simulink model "chris_3R_hsv_all_primitives"  (R2024b)
settings: Solver=FixedStepDiscrete  StartTime=0.0  StopTime=30  FixedStep=0.1  MaxStep=0.1  RelTol=1e-3
libraries: neural x110, realtime_pacer_lib x1, simulink x1
(part 2 of 7)

== system chris_3R_hsv_all_primitives/Cluster_Controller_HSV_steepest_descent/3_robot HSV to vector ==
  Sat : Inport
  Robot_1_pose : Inport  Port=2
  robot_2_pose : Inport  Port=3
  robot_3_pose : Inport  Port=4
  Constant2 : Constant  Value=0
  Demux{,1..3} (4 alike) : Demux  Outputs=3
  Desired_velocities_new_primitve : ToWorkspace  VariableName=desired_velocities_gradient_descent  SampleTime=-1
  MATLAB Function : MATLAB Function  TreatAsAtomicUnit=on
  Scope : Scope  NumInputPorts=2
  Scope1 : Scope  NumInputPorts=2
  Scope2 : Scope  NumInputPorts=2
  Vector Concatenate : Concatenate  NumInputs=3
  y_velocity : Outport
  x_velocity : Outport  Port=2
  th_c velocity : Outport  Port=3
  wires:
  Vector Concatenate/1 -> Desired_velocities_new_primitve/1
  Constant2/1 -> th_c velocity/1, Vector Concatenate/3
  Sat/1 -> Demux/1
  Robot_1_pose/1 -> Demux1/1
  robot_2_pose/1 -> Demux2/1
  robot_3_pose/1 -> Demux3/1
  Demux1/1 -> Scope1/1, MATLAB Function/1(x1)
  Demux1/2 -> MATLAB Function/2(y1), Scope1/2
  Demux/1 -> Scope2/1, MATLAB Function/3(z1)
  Demux2/1 -> MATLAB Function/4(x2)
  Demux2/2 -> MATLAB Function/5(y2)
  Demux/2 -> Scope2/2, MATLAB Function/6(z2)
  Demux3/1 -> MATLAB Function/7(x3)
  Demux3/2 -> MATLAB Function/8(y3)
  Demux/3 -> MATLAB Function/9(z3)
  MATLAB Function/1(x) -> Scope/1, x_velocity/1, Vector Concatenate/1
  MATLAB Function/2(y) -> Scope/2, y_velocity/1, Vector Concatenate/2

== system chris_3R_hsv_all_primitives/Cluster_Controller_HSV_steepest_descent/formation_error ==
  a : Inport
  b : Inport  Port=2
  c : Inport  Port=3
  a,b,c desired : Inport  Port=4
  Demux7 : Demux  Outputs=3
  Sum3 : Sum  Inputs=-+
  Sum4 : Sum  Inputs=-+
  Sum5 : Sum  Inputs=-+
  Out4 : Outport
  Out5 : Outport  Port=2
  Out6 : Outport  Port=3
  wires:
  Sum3/1 -> Out4/1
  Demux7/3 -> Sum5/2
  a,b,c desired/1 -> Demux7/1
  Demux7/1 -> Sum3/2
  b/1 -> Sum4/1
  Demux7/2 -> Sum4/2
  c/1 -> Sum5/1
  Sum4/1 -> Out5/1
  Sum5/1 -> Out6/1
  a/1 -> Sum3/1

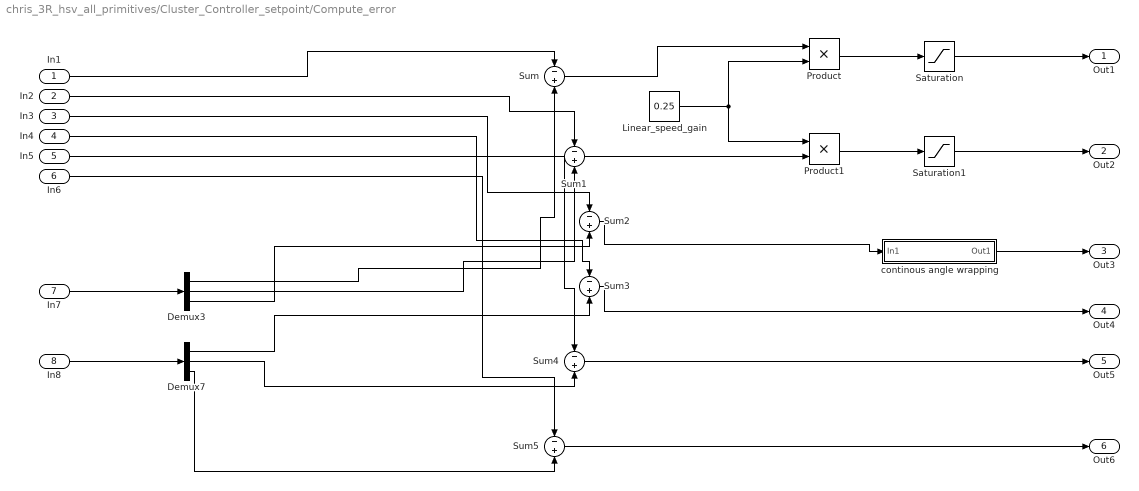
== system chris_3R_hsv_all_primitives/Cluster_Controller_setpoint/Compute_error ==
  In1 : Inport
  In2 : Inport  Port=2
  In3 : Inport  Port=3
  In4 : Inport  Port=4
  In5 : Inport  Port=5
  In6 : Inport  Port=6
  In7 : Inport  Port=7
  In8 : Inport  Port=8
  Demux3 : Demux  Outputs=3
  Demux7 : Demux  Outputs=3
  Linear_speed_gain : Constant  Value=0.25
  Product : Product
  Product1 : Product
  Saturation : Saturate
  Saturation1 : Saturate
  Sum{,1..5} (6 alike) : Sum  Inputs=-+
  continous angle wrapping : Subsystem
  Out1 : Outport
  Out2 : Outport  Port=2
  Out3 : Outport  Port=3
  Out4 : Outport  Port=4
  Out5 : Outport  Port=5
  Out6 : Outport  Port=6
  wires:
  In3/1 -> Sum2/1
  Demux3/2 -> Sum1/2
  Sum3/1 -> Out4/1
  In2/1 -> Sum1/1
  Demux3/3 -> Sum2/2
  Demux7/3 -> Sum5/2
  In8/1 -> Demux7/1
  Demux7/1 -> Sum3/2
  In1/1 -> Sum/1
  In5/1 -> Sum4/1
  Demux7/2 -> Sum4/2
  In6/1 -> Sum5/1
  Sum4/1 -> Out5/1
  Sum5/1 -> Out6/1
  Demux3/1 -> Sum/2
  In4/1 -> Sum3/1
  In7/1 -> Demux3/1
  Sum2/1 -> continous angle wrapping/1(In1)
  continous angle wrapping/1(Out1) -> Out3/1
  Sum/1 -> Product/1
  Linear_speed_gain/1 -> Product/2, Product1/1
  Sum1/1 -> Product1/2
  Saturation/1 -> Out1/1
  Product/1 -> Saturation/1
  Product1/1 -> Saturation1/1
  Saturation1/1 -> Out2/1

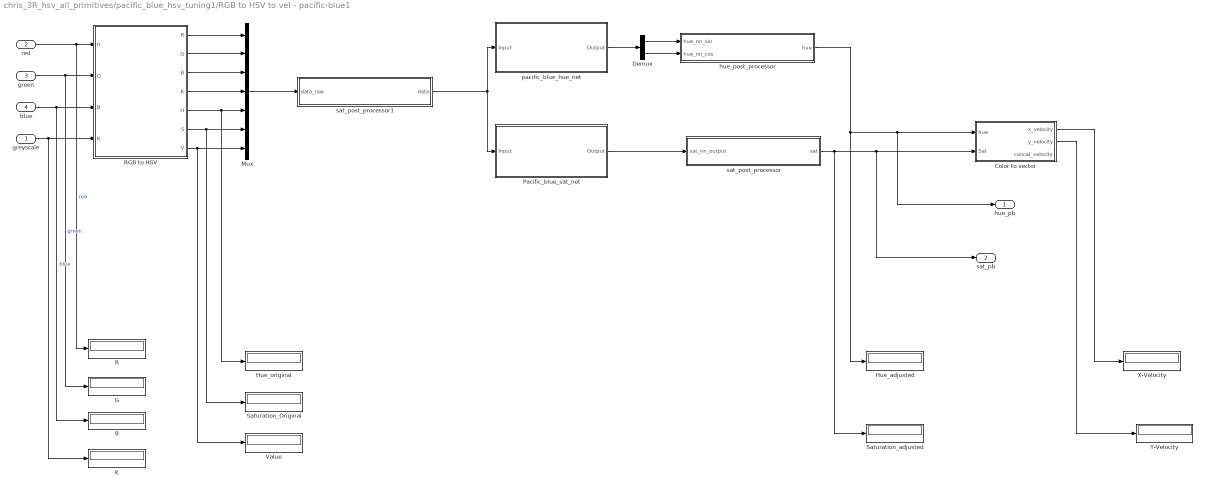
== system chris_3R_hsv_all_primitives/pacific_blue_hsv_tuning1/RGB to HSV to vel - pacific-blue1 ==
  greyscale : Inport
  red : Inport  Port=2
  green : Inport  Port=3
  blue : Inport  Port=4
  B : Display
  Color to vector : Subsystem
  Demux : Demux  Outputs=2
  G : Display
  Hue_adjusted : Display
  Hue_original : Display
  K : Display
  Mux : Mux  Inputs=7
  Pacific_blue_sat_net : Subsystem
      mask help: Feed-Forward Neural Network
      mask Display: e = 0.06;c1 = [120 150 230]/255;c2 = ([120 150 230]+0)/383;c3 = ([120 150 230]+128)/383;patch([0 1 1 0],[0 0 1 1],c1);patch([0 1 1 1-e 1-e 0+e],[0 0 1 1-e 0+e 0+e],c2);patch([0 0 1 1-e 0+e 0+e],[0 1 1 1-e 1-e 0+e],c3);plot([0 1 1 0 0],[0 0 1 1 0]);fprintf('NNET');port_label('input',1,' Input');port_label('output',1,'Output ');
  R : Display
  RGB to HSV : MATLAB Function  TreatAsAtomicUnit=on
  Saturation_Original : Display
  Saturation_adjusted : Display
  Value : Display
  X-Velocity : Display
  "Y-Velocity " : Display
  hue_post_processor : MATLAB Function  TreatAsAtomicUnit=on
  pacific_blue_hue_net : Subsystem
      mask help: Feed-Forward Neural Network
      mask Display: e = 0.06;c1 = [120 150 230]/255;c2 = ([120 150 230]+0)/383;c3 = ([120 150 230]+128)/383;patch([0 1 1 0],[0 0 1 1],c1);patch([0 1 1 1-e 1-e 0+e],[0 0 1 1-e 0+e 0+e],c2);patch([0 0 1 1-e 0+e 0+e],[0 1 1 1-e 1-e 0+e],c3);plot([0 1 1 0 0],[0 0 1 1 0]);fprintf('NNET');port_label('input',1,' Input');port_label('output',1,'Output ');
  sat_post_processor : MATLAB Function  TreatAsAtomicUnit=on
  sat_post_processor1 : MATLAB Function  TreatAsAtomicUnit=on
  hue_pb : Outport
  sat_pb : Outport  Port=2
  wires:
  red/1 -> R/1, RGB to HSV/1("R ")  "red"
  green/1 -> G/1, RGB to HSV/2("G ")  "green"
  blue/1 -> B/1, RGB to HSV/3("B ")  "blue"
  greyscale/1 -> K/1, RGB to HSV/4("K ")
  RGB to HSV/7(V) -> Value/1, Mux/7
  RGB to HSV/6(S) -> Saturation_Original/1, Mux/6
  RGB to HSV/5(H) -> Hue_original/1, Mux/5
  RGB to HSV/4(K) -> Mux/4
  RGB to HSV/3(B) -> Mux/3
  RGB to HSV/2(G) -> Mux/2
  RGB to HSV/1(R) -> Mux/1
  Pacific_blue_sat_net/1(Output) -> sat_post_processor/1(sat_nn_output)
  hue_post_processor/1(hue) -> Hue_adjusted/1, Color to vector/1(hue), hue_pb/1
  sat_post_processor/1(sat) -> Saturation_adjusted/1, Color to vector/2(Sat), sat_pb/1
  Color to vector/1(x_velocity) -> X-Velocity/1
  Color to vector/2(y_velocity) -> "Y-Velocity "/1
  pacific_blue_hue_net/1(Output) -> Demux/1
  Demux/1 -> hue_post_processor/1(hue_nn_sin)
  Demux/2 -> hue_post_processor/2(hue_nn_cos)
  sat_post_processor1/1(data) -> pacific_blue_hue_net/1(Input), Pacific_blue_sat_net/1(Input)
  Mux/1 -> sat_post_processor1/1(data_raw)

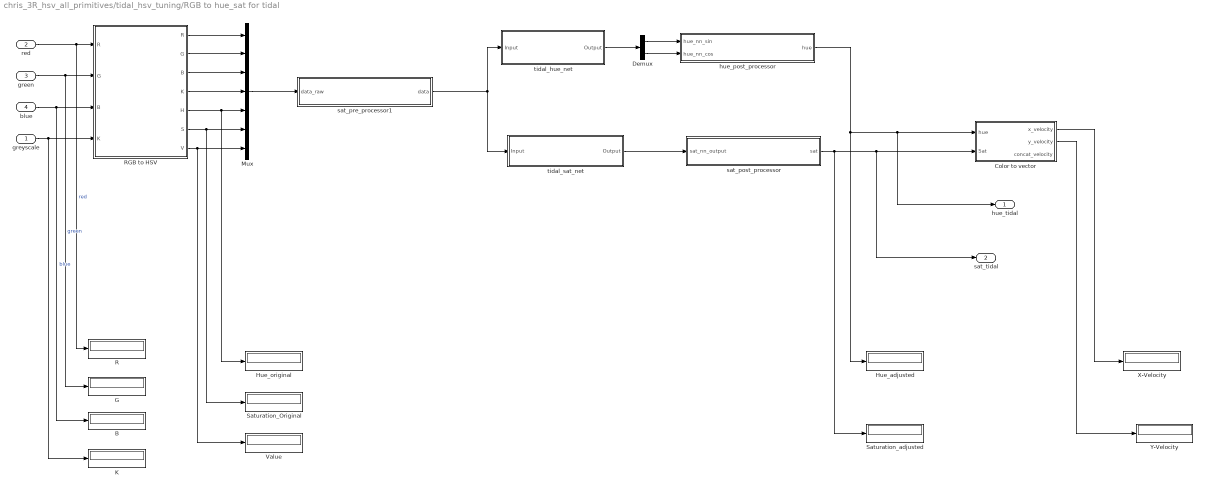
== system chris_3R_hsv_all_primitives/tidal_hsv_tuning/RGB to hue_sat for tidal ==
  greyscale : Inport
  red : Inport  Port=2
  green : Inport  Port=3
  blue : Inport  Port=4
  B : Display
  Color to vector : Subsystem
  Demux : Demux  Outputs=2
  G : Display
  Hue_adjusted : Display
  Hue_original : Display
  K : Display
  Mux : Mux  Inputs=7
  R : Display
  RGB to HSV : MATLAB Function  TreatAsAtomicUnit=on
  Saturation_Original : Display
  Saturation_adjusted : Display
  Value : Display
  X-Velocity : Display
  "Y-Velocity " : Display
  hue_post_processor : MATLAB Function  TreatAsAtomicUnit=on
  sat_post_processor : MATLAB Function  TreatAsAtomicUnit=on
  sat_pre_processor1 : MATLAB Function  TreatAsAtomicUnit=on
  tidal_hue_net : Subsystem
      mask help: Feed-Forward Neural Network
      mask Display: e = 0.06;c1 = [120 150 230]/255;c2 = ([120 150 230]+0)/383;c3 = ([120 150 230]+128)/383;patch([0 1 1 0],[0 0 1 1],c1);patch([0 1 1 1-e 1-e 0+e],[0 0 1 1-e 0+e 0+e],c2);patch([0 0 1 1-e 0+e 0+e],[0 1 1 1-e 1-e 0+e],c3);plot([0 1 1 0 0],[0 0 1 1 0]);fprintf('NNET');port_label('input',1,' Input');port_label('output',1,'Output ');
  tidal_sat_net : Subsystem
      mask help: Feed-Forward Neural Network
      mask Display: e = 0.06;c1 = [120 150 230]/255;c2 = ([120 150 230]+0)/383;c3 = ([120 150 230]+128)/383;patch([0 1 1 0],[0 0 1 1],c1);patch([0 1 1 1-e 1-e 0+e],[0 0 1 1-e 0+e 0+e],c2);patch([0 0 1 1-e 0+e 0+e],[0 1 1 1-e 1-e 0+e],c3);plot([0 1 1 0 0],[0 0 1 1 0]);fprintf('NNET');port_label('input',1,' Input');port_label('output',1,'Output ');
  hue_tidal : Outport
  sat_tidal : Outport  Port=2
  wires:
  Mux/1 -> sat_pre_processor1/1(data_raw)
  sat_pre_processor1/1(data) -> tidal_sat_net/1(Input), tidal_hue_net/1(Input)
  Demux/2 -> hue_post_processor/2(hue_nn_cos)
  Demux/1 -> hue_post_processor/1(hue_nn_sin)
  tidal_hue_net/1(Output) -> Demux/1
  Color to vector/2(y_velocity) -> "Y-Velocity "/1
  Color to vector/1(x_velocity) -> X-Velocity/1
  sat_post_processor/1(sat) -> sat_tidal/1, Color to vector/2(Sat), Saturation_adjusted/1
  hue_post_processor/1(hue) -> hue_tidal/1, Color to vector/1(hue), Hue_adjusted/1
  tidal_sat_net/1(Output) -> sat_post_processor/1(sat_nn_output)
  RGB to HSV/1(R) -> Mux/1
  RGB to HSV/2(G) -> Mux/2
  RGB to HSV/3(B) -> Mux/3
  RGB to HSV/4(K) -> Mux/4
  RGB to HSV/5(H) -> Mux/5, Hue_original/1
  RGB to HSV/6(S) -> Mux/6, Saturation_Original/1
  RGB to HSV/7(V) -> Mux/7, Value/1
  greyscale/1 -> RGB to HSV/4("K "), K/1
  blue/1 -> RGB to HSV/3("B "), B/1  "blue"
  green/1 -> RGB to HSV/2("G "), G/1  "green"
  red/1 -> RGB to HSV/1("R "), R/1  "red"

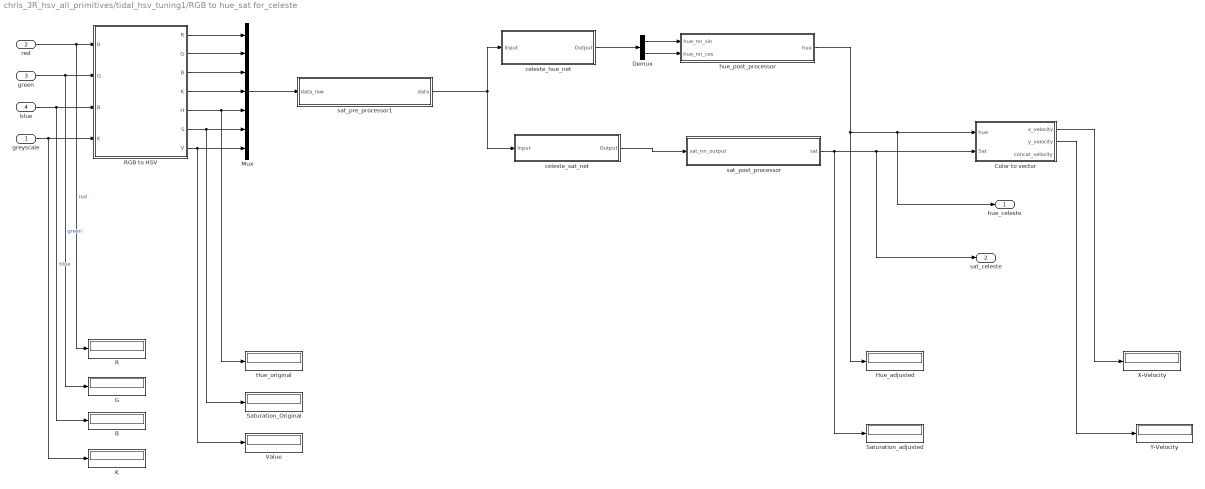
== system chris_3R_hsv_all_primitives/tidal_hsv_tuning1/RGB to hue_sat for_celeste ==
  greyscale : Inport
  red : Inport  Port=2
  green : Inport  Port=3
  blue : Inport  Port=4
  B : Display
  Color to vector : Subsystem
  Demux : Demux  Outputs=2
  G : Display
  Hue_adjusted : Display
  Hue_original : Display
  K : Display
  Mux : Mux  Inputs=7
  R : Display
  RGB to HSV : MATLAB Function  TreatAsAtomicUnit=on
  Saturation_Original : Display
  Saturation_adjusted : Display
  Value : Display
  X-Velocity : Display
  "Y-Velocity " : Display
  celeste_hue_net : Subsystem
      mask help: Feed-Forward Neural Network
      mask Display: e = 0.06;c1 = [120 150 230]/255;c2 = ([120 150 230]+0)/383;c3 = ([120 150 230]+128)/383;patch([0 1 1 0],[0 0 1 1],c1);patch([0 1 1 1-e 1-e 0+e],[0 0 1 1-e 0+e 0+e],c2);patch([0 0 1 1-e 0+e 0+e],[0 1 1 1-e 1-e 0+e],c3);plot([0 1 1 0 0],[0 0 1 1 0]);fprintf('NNET');port_label('input',1,' Input');port_label('output',1,'Output ');
  celeste_sat_net : Subsystem
      mask help: Feed-Forward Neural Network
      mask Display: e = 0.06;c1 = [120 150 230]/255;c2 = ([120 150 230]+0)/383;c3 = ([120 150 230]+128)/383;patch([0 1 1 0],[0 0 1 1],c1);patch([0 1 1 1-e 1-e 0+e],[0 0 1 1-e 0+e 0+e],c2);patch([0 0 1 1-e 0+e 0+e],[0 1 1 1-e 1-e 0+e],c3);plot([0 1 1 0 0],[0 0 1 1 0]);fprintf('NNET');port_label('input',1,' Input');port_label('output',1,'Output ');
  hue_post_processor : MATLAB Function  TreatAsAtomicUnit=on
  sat_post_processor : MATLAB Function  TreatAsAtomicUnit=on
  sat_pre_processor1 : MATLAB Function  TreatAsAtomicUnit=on
  hue_celeste : Outport
  sat_celeste : Outport  Port=2
  wires:
  Mux/1 -> sat_pre_processor1/1(data_raw)
  sat_pre_processor1/1(data) -> celeste_sat_net/1(Input), celeste_hue_net/1(Input)
  Demux/2 -> hue_post_processor/2(hue_nn_cos)
  Demux/1 -> hue_post_processor/1(hue_nn_sin)
  celeste_hue_net/1(Output) -> Demux/1
  Color to vector/2(y_velocity) -> "Y-Velocity "/1
  Color to vector/1(x_velocity) -> X-Velocity/1
  sat_post_processor/1(sat) -> sat_celeste/1, Color to vector/2(Sat), Saturation_adjusted/1
  hue_post_processor/1(hue) -> hue_celeste/1, Color to vector/1(hue), Hue_adjusted/1
  celeste_sat_net/1(Output) -> sat_post_processor/1(sat_nn_output)
  RGB to HSV/1(R) -> Mux/1
  RGB to HSV/2(G) -> Mux/2
  RGB to HSV/3(B) -> Mux/3
  RGB to HSV/4(K) -> Mux/4
  RGB to HSV/5(H) -> Mux/5, Hue_original/1
  RGB to HSV/6(S) -> Mux/6, Saturation_Original/1
  RGB to HSV/7(V) -> Mux/7, Value/1
  greyscale/1 -> RGB to HSV/4("K "), K/1
  blue/1 -> RGB to HSV/3("B "), B/1  "blue"
  green/1 -> RGB to HSV/2("G "), G/1  "green"
  red/1 -> RGB to HSV/1("R "), R/1  "red"

== system chris_3R_hsv_all_primitives/Cluster_Controller_HSV_direction_and_mag_follower/3_robot HSV to vector/Average_Saturation ==
  In1 : Inport
  Constant : Constant  Value=1/3
  Demux : Demux  Outputs=3
  Product7 : Product
  Sum1 : Sum  Inputs=|+++
  Out1 : Outport
  wires:
  Sum1/1 -> Product7/1
  Demux/3 -> Sum1/3
  Product7/1 -> Out1/1
  Demux/1 -> Sum1/1
  In1/1 -> Demux/1
  Demux/2 -> Sum1/2
  Constant/1 -> Product7/2

== system chris_3R_hsv_all_primitives/Cluster_Controller_HSV_direction_and_mag_follower/3_robot HSV to vector/Saturation_clipped_and_rescaled ==
  In1 : Inport
  Product7 : Product
  Saturation : Saturate  UpperLimit=1  LowerLimit=0.05
  Sum : Sum  Inputs=|+-
  clipped : Constant  Value=0.3
  rescale : Constant  Value=1.42857
  Out1 : Outport
  wires:
  clipped/1 -> Sum/2
  Saturation/1 -> Out1/1
  In1/1 -> Sum/1
  Product7/1 -> Saturation/1
  rescale/1 -> Product7/2
  Sum/1 -> Product7/1

== system chris_3R_hsv_all_primitives/Cluster_Controller_setpoint/Compute_error/continous angle wrapping ==
  In1 : Inport
  Constant : Constant  Value=pi
  Constant1 : Constant  Value=2*pi
  Math Function : Math  Operator=mod  SignedPower=on
  Sum6 : Sum
  Sum7 : Sum  Inputs=-+
  Out1 : Outport
  wires:
  In1/1 -> Sum6/2
  Math Function/1 -> Sum7/2
  Constant/1 -> Sum7/1, Sum6/1
  Sum6/1 -> Math Function/1
  Constant1/1 -> Math Function/2
  Sum7/1 -> Out1/1

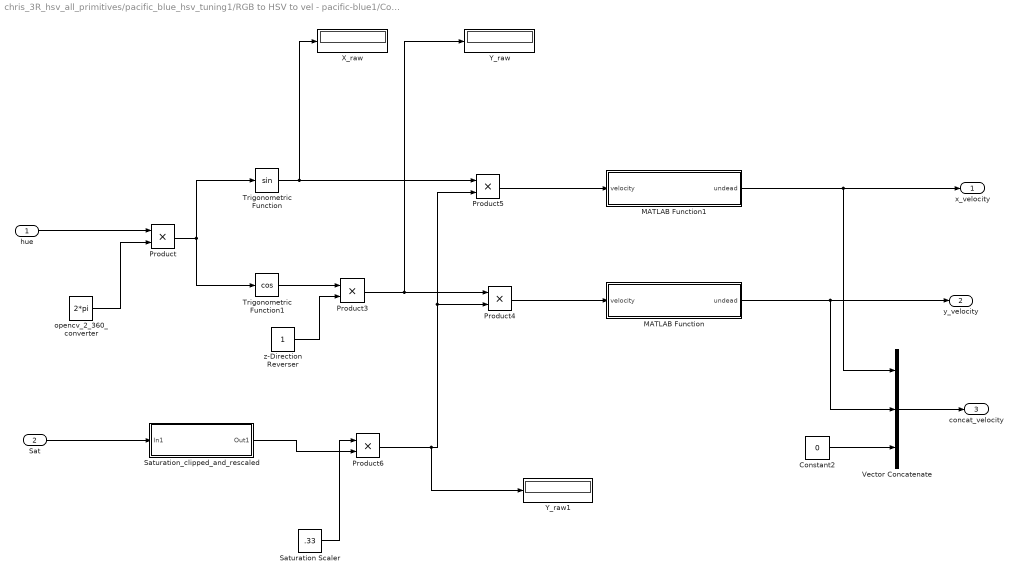
== system chris_3R_hsv_all_primitives/pacific_blue_hsv_tuning1/RGB to HSV to vel - pacific-blue1/Color to vector ==
  hue : Inport
  Sat : Inport  Port=2
  Constant2 : Constant  Value=0
  MATLAB Function : MATLAB Function  TreatAsAtomicUnit=on
  MATLAB Function1 : MATLAB Function  TreatAsAtomicUnit=on
  Product{,3..6} (5 alike) : Product
  Saturation Scaler : Constant  Value=.33
  Saturation_clipped_and_rescaled : Subsystem
  Trigonometric Function : Trigonometry
  Trigonometric Function1 : Trigonometry  Operator=cos
  Vector Concatenate : Concatenate  NumInputs=3
  X_raw : Display
  Y_raw : Display
  Y_raw1 : Display
  opencv_2_360_converter : Constant  Value=2*pi
  z-Direction Reverser : Constant
  x_velocity : Outport
  y_velocity : Outport  Port=2
  concat_velocity : Outport  Port=3
  wires:
  Trigonometric Function/1 -> Product5/1, X_raw/1
  opencv_2_360_converter/1 -> Product/2
  Product/1 -> Trigonometric Function1/1, Trigonometric Function/1
  Trigonometric Function1/1 -> Product3/1
  hue/1 -> Product/1
  Vector Concatenate/1 -> concat_velocity/1
  z-Direction Reverser/1 -> Product3/2
  Product3/1 -> Y_raw/1, Product4/1
  Constant2/1 -> Vector Concatenate/3
  Product6/1 -> Y_raw1/1, Product4/2, Product5/2
  Sat/1 -> Saturation_clipped_and_rescaled/1(In1)
  Product5/1 -> MATLAB Function1/1(velocity)
  MATLAB Function1/1(undead) -> Vector Concatenate/1, x_velocity/1
  MATLAB Function/1(undead) -> y_velocity/1, Vector Concatenate/2
  Product4/1 -> MATLAB Function/1(velocity)
  Saturation Scaler/1 -> Product6/1
  Saturation_clipped_and_rescaled/1(Out1) -> Product6/2

== system chris_3R_hsv_all_primitives/pacific_blue_hsv_tuning1/RGB to HSV to vel - pacific-blue1/Pacific_blue_sat_net ==
  Input : Inport  PortDimensions=7
      mask Display: e = 0.06;c1 = [120 230 180]/255;c2 = ([120 230 180]+0)/(256+128);c3 = ([120 230 180]+128)/(256+128);patch([0 1 1 0],[0 0 1 1],c1);patch([0 1 1 1-e 1-e 0+e],[0 0 1 1-e 0+e 0+e],c2);patch([0 0 1 1-e 0+e 0+e],[0 1 1 1-e 1-e 0+e],c3);plot([0 1 1 0 0],[0 0 1 1 0]);
  Layer 1 : Subsystem
      mask Display: e = 0.06;c1 = [120 150 230]/255;c2 = ([120 150 230]+0)/383;c3 = ([120 150 230]+128)/383;patch([0 1 1 0],[0 0 1 1],c1);patch([0 1 1 1-e 1-e 0+e],[0 0 1 1-e 0+e 0+e],c2);patch([0 0 1 1-e 0+e 0+e],[0 1 1 1-e 1-e 0+e],c3);plot([0 1 1 0 0],[0 0 1 1 0]);
  Layer 2 : Subsystem
      mask Display: e = 0.06;c1 = [120 150 230]/255;c2 = ([120 150 230]+0)/383;c3 = ([120 150 230]+128)/383;patch([0 1 1 0],[0 0 1 1],c1);patch([0 1 1 1-e 1-e 0+e],[0 0 1 1-e 0+e 0+e],c2);patch([0 0 1 1-e 0+e 0+e],[0 1 1 1-e 1-e 0+e],c3);plot([0 1 1 0 0],[0 0 1 1 0]);
  Layer 3 : Subsystem
      mask Display: e = 0.06;c1 = [120 150 230]/255;c2 = ([120 150 230]+0)/383;c3 = ([120 150 230]+128)/383;patch([0 1 1 0],[0 0 1 1],c1);patch([0 1 1 1-e 1-e 0+e],[0 0 1 1-e 0+e 0+e],c2);patch([0 0 1 1-e 0+e 0+e],[0 1 1 1-e 1-e 0+e],c3);plot([0 1 1 0 0],[0 0 1 1 0]);
  Layer 4 : Subsystem
      mask Display: e = 0.06;c1 = [120 150 230]/255;c2 = ([120 150 230]+0)/383;c3 = ([120 150 230]+128)/383;patch([0 1 1 0],[0 0 1 1],c1);patch([0 1 1 1-e 1-e 0+e],[0 0 1 1-e 0+e 0+e],c2);patch([0 0 1 1-e 0+e 0+e],[0 1 1 1-e 1-e 0+e],c3);plot([0 1 1 0 0],[0 0 1 1 0]);
  Process Input 1 : Subsystem
      mask Display: e = 0.06;c1 = [120 150 230]/255;c2 = ([120 150 230]+0)/383;c3 = ([120 150 230]+128)/383;patch([0 1 1 0],[0 0 1 1],c1);patch([0 1 1 1-e 1-e 0+e],[0 0 1 1-e 0+e 0+e],c2);patch([0 0 1 1-e 0+e 0+e],[0 1 1 1-e 1-e 0+e],c3);plot([0 1 1 0 0],[0 0 1 1 0]);
  Process Output 1 : Subsystem
      mask Display: e = 0.06;c1 = [120 150 230]/255;c2 = ([120 150 230]+0)/383;c3 = ([120 150 230]+128)/383;patch([0 1 1 0],[0 0 1 1],c1);patch([0 1 1 1-e 1-e 0+e],[0 0 1 1-e 0+e 0+e],c2);patch([0 0 1 1-e 0+e 0+e],[0 1 1 1-e 1-e 0+e],c3);plot([0 1 1 0 0],[0 0 1 1 0]);
  Output : Outport  InitialOutput=0
      mask Display: e = 0.06;c1 = [120 230 180]/255;c2 = ([120 230 180]+0)/(256+128);c3 = ([120 230 180]+128)/(256+128);patch([0 1 1 0],[0 0 1 1],c1);patch([0 1 1 1-e 1-e 0+e],[0 0 1 1-e 0+e 0+e],c2);patch([0 0 1 1-e 0+e 0+e],[0 1 1 1-e 1-e 0+e],c3);plot([0 1 1 0 0],[0 0 1 1 0]);
  wires:
  Layer 4/1("a{4}") -> Process Output 1/1(a)
  [feedback3] -> Layer 4/1("a{3} ")
  Layer 3/1("a{3}") -> [feedback3]
  [feedback2] -> Layer 3/1("a{2} ")
  Layer 2/1("a{2}") -> [feedback2]
  [feedback1] -> Layer 2/1("a{1} ")
  Layer 1/1("a{1}") -> [feedback1]
  Process Input 1/1(p) -> Layer 1/1("p{1}")
  Process Output 1/1(y) -> Output/1
  Input/1 -> Process Input 1/1(x)

== system chris_3R_hsv_all_primitives/pacific_blue_hsv_tuning1/RGB to HSV to vel - pacific-blue1/pacific_blue_hue_net ==
  Input : Inport  PortDimensions=7
      mask Display: e = 0.06;c1 = [120 230 180]/255;c2 = ([120 230 180]+0)/(256+128);c3 = ([120 230 180]+128)/(256+128);patch([0 1 1 0],[0 0 1 1],c1);patch([0 1 1 1-e 1-e 0+e],[0 0 1 1-e 0+e 0+e],c2);patch([0 0 1 1-e 0+e 0+e],[0 1 1 1-e 1-e 0+e],c3);plot([0 1 1 0 0],[0 0 1 1 0]);
  Layer 1 : Subsystem
      mask Display: e = 0.06;c1 = [120 150 230]/255;c2 = ([120 150 230]+0)/383;c3 = ([120 150 230]+128)/383;patch([0 1 1 0],[0 0 1 1],c1);patch([0 1 1 1-e 1-e 0+e],[0 0 1 1-e 0+e 0+e],c2);patch([0 0 1 1-e 0+e 0+e],[0 1 1 1-e 1-e 0+e],c3);plot([0 1 1 0 0],[0 0 1 1 0]);
  Layer 2 : Subsystem
      mask Display: e = 0.06;c1 = [120 150 230]/255;c2 = ([120 150 230]+0)/383;c3 = ([120 150 230]+128)/383;patch([0 1 1 0],[0 0 1 1],c1);patch([0 1 1 1-e 1-e 0+e],[0 0 1 1-e 0+e 0+e],c2);patch([0 0 1 1-e 0+e 0+e],[0 1 1 1-e 1-e 0+e],c3);plot([0 1 1 0 0],[0 0 1 1 0]);
  Layer 3 : Subsystem
      mask Display: e = 0.06;c1 = [120 150 230]/255;c2 = ([120 150 230]+0)/383;c3 = ([120 150 230]+128)/383;patch([0 1 1 0],[0 0 1 1],c1);patch([0 1 1 1-e 1-e 0+e],[0 0 1 1-e 0+e 0+e],c2);patch([0 0 1 1-e 0+e 0+e],[0 1 1 1-e 1-e 0+e],c3);plot([0 1 1 0 0],[0 0 1 1 0]);
  Process Input 1 : Subsystem
      mask Display: e = 0.06;c1 = [120 150 230]/255;c2 = ([120 150 230]+0)/383;c3 = ([120 150 230]+128)/383;patch([0 1 1 0],[0 0 1 1],c1);patch([0 1 1 1-e 1-e 0+e],[0 0 1 1-e 0+e 0+e],c2);patch([0 0 1 1-e 0+e 0+e],[0 1 1 1-e 1-e 0+e],c3);plot([0 1 1 0 0],[0 0 1 1 0]);
  Process Output 1 : Subsystem
      mask Display: e = 0.06;c1 = [120 150 230]/255;c2 = ([120 150 230]+0)/383;c3 = ([120 150 230]+128)/383;patch([0 1 1 0],[0 0 1 1],c1);patch([0 1 1 1-e 1-e 0+e],[0 0 1 1-e 0+e 0+e],c2);patch([0 0 1 1-e 0+e 0+e],[0 1 1 1-e 1-e 0+e],c3);plot([0 1 1 0 0],[0 0 1 1 0]);
  Output : Outport  InitialOutput=[0;0]
      mask Display: e = 0.06;c1 = [120 230 180]/255;c2 = ([120 230 180]+0)/(256+128);c3 = ([120 230 180]+128)/(256+128);patch([0 1 1 0],[0 0 1 1],c1);patch([0 1 1 1-e 1-e 0+e],[0 0 1 1-e 0+e 0+e],c2);patch([0 0 1 1-e 0+e 0+e],[0 1 1 1-e 1-e 0+e],c3);plot([0 1 1 0 0],[0 0 1 1 0]);
  wires:
  Input/1 -> Process Input 1/1(x)
  Process Output 1/1(y) -> Output/1
  Process Input 1/1(p) -> Layer 1/1("p{1}")
  Layer 1/1("a{1}") -> [feedback1]
  [feedback1] -> Layer 2/1("a{1} ")
  Layer 2/1("a{2}") -> [feedback2]
  [feedback2] -> Layer 3/1("a{2} ")
  Layer 3/1("a{3}") -> Process Output 1/1(a)

== system chris_3R_hsv_all_primitives/tidal_hsv_tuning/RGB to hue_sat for tidal/Color to vector ==
  hue : Inport
  Sat : Inport  Port=2
  Constant2 : Constant  Value=0
  MATLAB Function : MATLAB Function  TreatAsAtomicUnit=on
  MATLAB Function1 : MATLAB Function  TreatAsAtomicUnit=on
  Product{,3..6} (5 alike) : Product
  Saturation Scaler : Constant  Value=.33
  Saturation_clipped_and_rescaled : Subsystem
  Trigonometric Function : Trigonometry
  Trigonometric Function1 : Trigonometry  Operator=cos
  Vector Concatenate : Concatenate  NumInputs=3
  X_raw : Display
  Y_raw : Display
  Y_raw1 : Display
  opencv_2_360_converter : Constant  Value=2*pi
  z-Direction Reverser : Constant
  x_velocity : Outport
  y_velocity : Outport  Port=2
  concat_velocity : Outport  Port=3
  wires:
  Saturation_clipped_and_rescaled/1(Out1) -> Product6/2
  Saturation Scaler/1 -> Product6/1
  Product4/1 -> MATLAB Function/1(velocity)
  MATLAB Function/1(undead) -> Vector Concatenate/2, y_velocity/1
  MATLAB Function1/1(undead) -> x_velocity/1, Vector Concatenate/1
  Product5/1 -> MATLAB Function1/1(velocity)
  Sat/1 -> Saturation_clipped_and_rescaled/1(In1)
  Product6/1 -> Product5/2, Product4/2, Y_raw1/1
  Constant2/1 -> Vector Concatenate/3
  Product3/1 -> Product4/1, Y_raw/1
  z-Direction Reverser/1 -> Product3/2
  Vector Concatenate/1 -> concat_velocity/1
  hue/1 -> Product/1
  Trigonometric Function1/1 -> Product3/1
  Product/1 -> Trigonometric Function/1, Trigonometric Function1/1
  opencv_2_360_converter/1 -> Product/2
  Trigonometric Function/1 -> X_raw/1, Product5/1

== system chris_3R_hsv_all_primitives/tidal_hsv_tuning/RGB to hue_sat for tidal/tidal_hue_net ==
  Input : Inport  PortDimensions=7
      mask Display: e = 0.06;c1 = [120 230 180]/255;c2 = ([120 230 180]+0)/(256+128);c3 = ([120 230 180]+128)/(256+128);patch([0 1 1 0],[0 0 1 1],c1);patch([0 1 1 1-e 1-e 0+e],[0 0 1 1-e 0+e 0+e],c2);patch([0 0 1 1-e 0+e 0+e],[0 1 1 1-e 1-e 0+e],c3);plot([0 1 1 0 0],[0 0 1 1 0]);
  Layer 1 : Subsystem
      mask Display: e = 0.06;c1 = [120 150 230]/255;c2 = ([120 150 230]+0)/383;c3 = ([120 150 230]+128)/383;patch([0 1 1 0],[0 0 1 1],c1);patch([0 1 1 1-e 1-e 0+e],[0 0 1 1-e 0+e 0+e],c2);patch([0 0 1 1-e 0+e 0+e],[0 1 1 1-e 1-e 0+e],c3);plot([0 1 1 0 0],[0 0 1 1 0]);
  Layer 2 : Subsystem
      mask Display: e = 0.06;c1 = [120 150 230]/255;c2 = ([120 150 230]+0)/383;c3 = ([120 150 230]+128)/383;patch([0 1 1 0],[0 0 1 1],c1);patch([0 1 1 1-e 1-e 0+e],[0 0 1 1-e 0+e 0+e],c2);patch([0 0 1 1-e 0+e 0+e],[0 1 1 1-e 1-e 0+e],c3);plot([0 1 1 0 0],[0 0 1 1 0]);
  Layer 3 : Subsystem
      mask Display: e = 0.06;c1 = [120 150 230]/255;c2 = ([120 150 230]+0)/383;c3 = ([120 150 230]+128)/383;patch([0 1 1 0],[0 0 1 1],c1);patch([0 1 1 1-e 1-e 0+e],[0 0 1 1-e 0+e 0+e],c2);patch([0 0 1 1-e 0+e 0+e],[0 1 1 1-e 1-e 0+e],c3);plot([0 1 1 0 0],[0 0 1 1 0]);
  Process Input 1 : Subsystem
      mask Display: e = 0.06;c1 = [120 150 230]/255;c2 = ([120 150 230]+0)/383;c3 = ([120 150 230]+128)/383;patch([0 1 1 0],[0 0 1 1],c1);patch([0 1 1 1-e 1-e 0+e],[0 0 1 1-e 0+e 0+e],c2);patch([0 0 1 1-e 0+e 0+e],[0 1 1 1-e 1-e 0+e],c3);plot([0 1 1 0 0],[0 0 1 1 0]);
  Process Output 1 : Subsystem
      mask Display: e = 0.06;c1 = [120 150 230]/255;c2 = ([120 150 230]+0)/383;c3 = ([120 150 230]+128)/383;patch([0 1 1 0],[0 0 1 1],c1);patch([0 1 1 1-e 1-e 0+e],[0 0 1 1-e 0+e 0+e],c2);patch([0 0 1 1-e 0+e 0+e],[0 1 1 1-e 1-e 0+e],c3);plot([0 1 1 0 0],[0 0 1 1 0]);
  Output : Outport  InitialOutput=[0;0]
      mask Display: e = 0.06;c1 = [120 230 180]/255;c2 = ([120 230 180]+0)/(256+128);c3 = ([120 230 180]+128)/(256+128);patch([0 1 1 0],[0 0 1 1],c1);patch([0 1 1 1-e 1-e 0+e],[0 0 1 1-e 0+e 0+e],c2);patch([0 0 1 1-e 0+e 0+e],[0 1 1 1-e 1-e 0+e],c3);plot([0 1 1 0 0],[0 0 1 1 0]);
  wires:
  Input/1 -> Process Input 1/1(x)
  Process Output 1/1(y) -> Output/1
  Process Input 1/1(p) -> Layer 1/1("p{1}")
  Layer 1/1("a{1}") -> [feedback1]
  [feedback1] -> Layer 2/1("a{1} ")
  Layer 2/1("a{2}") -> [feedback2]
  [feedback2] -> Layer 3/1("a{2} ")
  Layer 3/1("a{3}") -> Process Output 1/1(a)

== system chris_3R_hsv_all_primitives/tidal_hsv_tuning/RGB to hue_sat for tidal/tidal_sat_net ==
  Input : Inport  PortDimensions=7
      mask Display: e = 0.06;c1 = [120 230 180]/255;c2 = ([120 230 180]+0)/(256+128);c3 = ([120 230 180]+128)/(256+128);patch([0 1 1 0],[0 0 1 1],c1);patch([0 1 1 1-e 1-e 0+e],[0 0 1 1-e 0+e 0+e],c2);patch([0 0 1 1-e 0+e 0+e],[0 1 1 1-e 1-e 0+e],c3);plot([0 1 1 0 0],[0 0 1 1 0]);
  Layer 1 : Subsystem
      mask Display: e = 0.06;c1 = [120 150 230]/255;c2 = ([120 150 230]+0)/383;c3 = ([120 150 230]+128)/383;patch([0 1 1 0],[0 0 1 1],c1);patch([0 1 1 1-e 1-e 0+e],[0 0 1 1-e 0+e 0+e],c2);patch([0 0 1 1-e 0+e 0+e],[0 1 1 1-e 1-e 0+e],c3);plot([0 1 1 0 0],[0 0 1 1 0]);
  Layer 2 : Subsystem
      mask Display: e = 0.06;c1 = [120 150 230]/255;c2 = ([120 150 230]+0)/383;c3 = ([120 150 230]+128)/383;patch([0 1 1 0],[0 0 1 1],c1);patch([0 1 1 1-e 1-e 0+e],[0 0 1 1-e 0+e 0+e],c2);patch([0 0 1 1-e 0+e 0+e],[0 1 1 1-e 1-e 0+e],c3);plot([0 1 1 0 0],[0 0 1 1 0]);
  Layer 3 : Subsystem
      mask Display: e = 0.06;c1 = [120 150 230]/255;c2 = ([120 150 230]+0)/383;c3 = ([120 150 230]+128)/383;patch([0 1 1 0],[0 0 1 1],c1);patch([0 1 1 1-e 1-e 0+e],[0 0 1 1-e 0+e 0+e],c2);patch([0 0 1 1-e 0+e 0+e],[0 1 1 1-e 1-e 0+e],c3);plot([0 1 1 0 0],[0 0 1 1 0]);
  Process Input 1 : Subsystem
      mask Display: e = 0.06;c1 = [120 150 230]/255;c2 = ([120 150 230]+0)/383;c3 = ([120 150 230]+128)/383;patch([0 1 1 0],[0 0 1 1],c1);patch([0 1 1 1-e 1-e 0+e],[0 0 1 1-e 0+e 0+e],c2);patch([0 0 1 1-e 0+e 0+e],[0 1 1 1-e 1-e 0+e],c3);plot([0 1 1 0 0],[0 0 1 1 0]);
  Process Output 1 : Subsystem
      mask Display: e = 0.06;c1 = [120 150 230]/255;c2 = ([120 150 230]+0)/383;c3 = ([120 150 230]+128)/383;patch([0 1 1 0],[0 0 1 1],c1);patch([0 1 1 1-e 1-e 0+e],[0 0 1 1-e 0+e 0+e],c2);patch([0 0 1 1-e 0+e 0+e],[0 1 1 1-e 1-e 0+e],c3);plot([0 1 1 0 0],[0 0 1 1 0]);
  Output : Outport  InitialOutput=0
      mask Display: e = 0.06;c1 = [120 230 180]/255;c2 = ([120 230 180]+0)/(256+128);c3 = ([120 230 180]+128)/(256+128);patch([0 1 1 0],[0 0 1 1],c1);patch([0 1 1 1-e 1-e 0+e],[0 0 1 1-e 0+e 0+e],c2);patch([0 0 1 1-e 0+e 0+e],[0 1 1 1-e 1-e 0+e],c3);plot([0 1 1 0 0],[0 0 1 1 0]);
  wires:
  Input/1 -> Process Input 1/1(x)
  Process Output 1/1(y) -> Output/1
  Process Input 1/1(p) -> Layer 1/1("p{1}")
  Layer 1/1("a{1}") -> [feedback1]
  [feedback1] -> Layer 2/1("a{1} ")
  Layer 2/1("a{2}") -> [feedback2]
  [feedback2] -> Layer 3/1("a{2} ")
  Layer 3/1("a{3}") -> Process Output 1/1(a)

== system chris_3R_hsv_all_primitives/tidal_hsv_tuning1/RGB to hue_sat for_celeste/Color to vector ==
  hue : Inport
  Sat : Inport  Port=2
  Constant2 : Constant  Value=0
  MATLAB Function : MATLAB Function  TreatAsAtomicUnit=on
  MATLAB Function1 : MATLAB Function  TreatAsAtomicUnit=on
  Product{,3..6} (5 alike) : Product
  Saturation Scaler : Constant  Value=.33
  Saturation_clipped_and_rescaled : Subsystem
  Trigonometric Function : Trigonometry
  Trigonometric Function1 : Trigonometry  Operator=cos
  Vector Concatenate : Concatenate  NumInputs=3
  X_raw : Display
  Y_raw : Display
  Y_raw1 : Display
  opencv_2_360_converter : Constant  Value=2*pi
  z-Direction Reverser : Constant
  x_velocity : Outport
  y_velocity : Outport  Port=2
  concat_velocity : Outport  Port=3
  wires:
  Saturation_clipped_and_rescaled/1(Out1) -> Product6/2
  Saturation Scaler/1 -> Product6/1
  Product4/1 -> MATLAB Function/1(velocity)
  MATLAB Function/1(undead) -> Vector Concatenate/2, y_velocity/1
  MATLAB Function1/1(undead) -> x_velocity/1, Vector Concatenate/1
  Product5/1 -> MATLAB Function1/1(velocity)
  Sat/1 -> Saturation_clipped_and_rescaled/1(In1)
  Product6/1 -> Product5/2, Product4/2, Y_raw1/1
  Constant2/1 -> Vector Concatenate/3
  Product3/1 -> Product4/1, Y_raw/1
  z-Direction Reverser/1 -> Product3/2
  Vector Concatenate/1 -> concat_velocity/1
  hue/1 -> Product/1
  Trigonometric Function1/1 -> Product3/1
  Product/1 -> Trigonometric Function/1, Trigonometric Function1/1
  opencv_2_360_converter/1 -> Product/2
  Trigonometric Function/1 -> X_raw/1, Product5/1

== system chris_3R_hsv_all_primitives/tidal_hsv_tuning1/RGB to hue_sat for_celeste/celeste_hue_net ==
  Input : Inport  PortDimensions=7
      mask Display: e = 0.06;c1 = [120 230 180]/255;c2 = ([120 230 180]+0)/(256+128);c3 = ([120 230 180]+128)/(256+128);patch([0 1 1 0],[0 0 1 1],c1);patch([0 1 1 1-e 1-e 0+e],[0 0 1 1-e 0+e 0+e],c2);patch([0 0 1 1-e 0+e 0+e],[0 1 1 1-e 1-e 0+e],c3);plot([0 1 1 0 0],[0 0 1 1 0]);
  Layer 1 : Subsystem
      mask Display: e = 0.06;c1 = [120 150 230]/255;c2 = ([120 150 230]+0)/383;c3 = ([120 150 230]+128)/383;patch([0 1 1 0],[0 0 1 1],c1);patch([0 1 1 1-e 1-e 0+e],[0 0 1 1-e 0+e 0+e],c2);patch([0 0 1 1-e 0+e 0+e],[0 1 1 1-e 1-e 0+e],c3);plot([0 1 1 0 0],[0 0 1 1 0]);
  Layer 2 : Subsystem
      mask Display: e = 0.06;c1 = [120 150 230]/255;c2 = ([120 150 230]+0)/383;c3 = ([120 150 230]+128)/383;patch([0 1 1 0],[0 0 1 1],c1);patch([0 1 1 1-e 1-e 0+e],[0 0 1 1-e 0+e 0+e],c2);patch([0 0 1 1-e 0+e 0+e],[0 1 1 1-e 1-e 0+e],c3);plot([0 1 1 0 0],[0 0 1 1 0]);
  Layer 3 : Subsystem
      mask Display: e = 0.06;c1 = [120 150 230]/255;c2 = ([120 150 230]+0)/383;c3 = ([120 150 230]+128)/383;patch([0 1 1 0],[0 0 1 1],c1);patch([0 1 1 1-e 1-e 0+e],[0 0 1 1-e 0+e 0+e],c2);patch([0 0 1 1-e 0+e 0+e],[0 1 1 1-e 1-e 0+e],c3);plot([0 1 1 0 0],[0 0 1 1 0]);
  Process Input 1 : Subsystem
      mask Display: e = 0.06;c1 = [120 150 230]/255;c2 = ([120 150 230]+0)/383;c3 = ([120 150 230]+128)/383;patch([0 1 1 0],[0 0 1 1],c1);patch([0 1 1 1-e 1-e 0+e],[0 0 1 1-e 0+e 0+e],c2);patch([0 0 1 1-e 0+e 0+e],[0 1 1 1-e 1-e 0+e],c3);plot([0 1 1 0 0],[0 0 1 1 0]);
  Process Output 1 : Subsystem
      mask Display: e = 0.06;c1 = [120 150 230]/255;c2 = ([120 150 230]+0)/383;c3 = ([120 150 230]+128)/383;patch([0 1 1 0],[0 0 1 1],c1);patch([0 1 1 1-e 1-e 0+e],[0 0 1 1-e 0+e 0+e],c2);patch([0 0 1 1-e 0+e 0+e],[0 1 1 1-e 1-e 0+e],c3);plot([0 1 1 0 0],[0 0 1 1 0]);
  Output : Outport  InitialOutput=[0;0]
      mask Display: e = 0.06;c1 = [120 230 180]/255;c2 = ([120 230 180]+0)/(256+128);c3 = ([120 230 180]+128)/(256+128);patch([0 1 1 0],[0 0 1 1],c1);patch([0 1 1 1-e 1-e 0+e],[0 0 1 1-e 0+e 0+e],c2);patch([0 0 1 1-e 0+e 0+e],[0 1 1 1-e 1-e 0+e],c3);plot([0 1 1 0 0],[0 0 1 1 0]);
  wires:
  Input/1 -> Process Input 1/1(x)
  Process Output 1/1(y) -> Output/1
  Process Input 1/1(p) -> Layer 1/1("p{1}")
  Layer 1/1("a{1}") -> [feedback1]
  [feedback1] -> Layer 2/1("a{1} ")
  Layer 2/1("a{2}") -> [feedback2]
  [feedback2] -> Layer 3/1("a{2} ")
  Layer 3/1("a{3}") -> Process Output 1/1(a)

== system chris_3R_hsv_all_primitives/tidal_hsv_tuning1/RGB to hue_sat for_celeste/celeste_sat_net ==
  Input : Inport  PortDimensions=7
      mask Display: e = 0.06;c1 = [120 230 180]/255;c2 = ([120 230 180]+0)/(256+128);c3 = ([120 230 180]+128)/(256+128);patch([0 1 1 0],[0 0 1 1],c1);patch([0 1 1 1-e 1-e 0+e],[0 0 1 1-e 0+e 0+e],c2);patch([0 0 1 1-e 0+e 0+e],[0 1 1 1-e 1-e 0+e],c3);plot([0 1 1 0 0],[0 0 1 1 0]);
  Layer 1 : Subsystem
      mask Display: e = 0.06;c1 = [120 150 230]/255;c2 = ([120 150 230]+0)/383;c3 = ([120 150 230]+128)/383;patch([0 1 1 0],[0 0 1 1],c1);patch([0 1 1 1-e 1-e 0+e],[0 0 1 1-e 0+e 0+e],c2);patch([0 0 1 1-e 0+e 0+e],[0 1 1 1-e 1-e 0+e],c3);plot([0 1 1 0 0],[0 0 1 1 0]);
  Layer 2 : Subsystem
      mask Display: e = 0.06;c1 = [120 150 230]/255;c2 = ([120 150 230]+0)/383;c3 = ([120 150 230]+128)/383;patch([0 1 1 0],[0 0 1 1],c1);patch([0 1 1 1-e 1-e 0+e],[0 0 1 1-e 0+e 0+e],c2);patch([0 0 1 1-e 0+e 0+e],[0 1 1 1-e 1-e 0+e],c3);plot([0 1 1 0 0],[0 0 1 1 0]);
  Layer 3 : Subsystem
      mask Display: e = 0.06;c1 = [120 150 230]/255;c2 = ([120 150 230]+0)/383;c3 = ([120 150 230]+128)/383;patch([0 1 1 0],[0 0 1 1],c1);patch([0 1 1 1-e 1-e 0+e],[0 0 1 1-e 0+e 0+e],c2);patch([0 0 1 1-e 0+e 0+e],[0 1 1 1-e 1-e 0+e],c3);plot([0 1 1 0 0],[0 0 1 1 0]);
  Process Input 1 : Subsystem
      mask Display: e = 0.06;c1 = [120 150 230]/255;c2 = ([120 150 230]+0)/383;c3 = ([120 150 230]+128)/383;patch([0 1 1 0],[0 0 1 1],c1);patch([0 1 1 1-e 1-e 0+e],[0 0 1 1-e 0+e 0+e],c2);patch([0 0 1 1-e 0+e 0+e],[0 1 1 1-e 1-e 0+e],c3);plot([0 1 1 0 0],[0 0 1 1 0]);
  Process Output 1 : Subsystem
      mask Display: e = 0.06;c1 = [120 150 230]/255;c2 = ([120 150 230]+0)/383;c3 = ([120 150 230]+128)/383;patch([0 1 1 0],[0 0 1 1],c1);patch([0 1 1 1-e 1-e 0+e],[0 0 1 1-e 0+e 0+e],c2);patch([0 0 1 1-e 0+e 0+e],[0 1 1 1-e 1-e 0+e],c3);plot([0 1 1 0 0],[0 0 1 1 0]);
  Output : Outport  InitialOutput=0
      mask Display: e = 0.06;c1 = [120 230 180]/255;c2 = ([120 230 180]+0)/(256+128);c3 = ([120 230 180]+128)/(256+128);patch([0 1 1 0],[0 0 1 1],c1);patch([0 1 1 1-e 1-e 0+e],[0 0 1 1-e 0+e 0+e],c2);patch([0 0 1 1-e 0+e 0+e],[0 1 1 1-e 1-e 0+e],c3);plot([0 1 1 0 0],[0 0 1 1 0]);
  wires:
  Input/1 -> Process Input 1/1(x)
  Process Output 1/1(y) -> Output/1
  Process Input 1/1(p) -> Layer 1/1("p{1}")
  Layer 1/1("a{1}") -> [feedback1]
  [feedback1] -> Layer 2/1("a{1} ")
  Layer 2/1("a{2}") -> [feedback2]
  [feedback2] -> Layer 3/1("a{2} ")
  Layer 3/1("a{3}") -> Process Output 1/1(a)

== system chris_3R_hsv_all_primitives/pacific_blue_hsv_tuning1/RGB to HSV to vel - pacific-blue1/Color to vector/Saturation_clipped_and_rescaled ==
  In1 : Inport
  Product7 : Product
  Saturation : Saturate  UpperLimit=1  LowerLimit=0.05
  Sum : Sum  Inputs=|+-
  clipped : Constant  Value=0.3
  rescale : Constant  Value=1.42857
  Out1 : Outport
  wires:
  clipped/1 -> Sum/2
  Saturation/1 -> Out1/1
  In1/1 -> Sum/1
  Product7/1 -> Saturation/1
  rescale/1 -> Product7/2
  Sum/1 -> Product7/1

== system chris_3R_hsv_all_primitives/pacific_blue_hsv_tuning1/RGB to HSV to vel - pacific-blue1/Pacific_blue_sat_net/Layer 1 ==
  "p{1}" : Inport  PortDimensions=7
      mask Display: e = 0.06;c1 = [120 230 180]/255;c2 = ([120 230 180]+0)/(256+128);c3 = ([120 230 180]+128)/(256+128);patch([0 1 1 0],[0 0 1 1],c1);patch([0 1 1 1-e 1-e 0+e],[0 0 1 1-e 0+e 0+e],c2);patch([0 0 1 1-e 0+e 0+e],[0 1 1 1-e 1-e 0+e],c3);plot([0 1 1 0 0],[0 0 1 1 0]);
  Delays 1 : Subsystem
      mask Display: e = 0.06;c1 = [120 150 230]/255;c2 = ([120 150 230]+0)/383;c3 = ([120 150 230]+128)/383;patch([0 1 1 0],[0 0 1 1],c1);patch([0 1 1 1-e 1-e 0+e],[0 0 1 1-e 0+e 0+e],c2);patch([0 0 1 1-e 0+e 0+e],[0 1 1 1-e 1-e 0+e],c3);plot([0 1 1 0 0],[0 0 1 1 0]);disp('0');
  "IW{1,1}" : Subsystem
      mask Display: e = 0.06;c1 = [120 150 230]/255;c2 = ([120 150 230]+0)/383;c3 = ([120 150 230]+128)/383;patch([0 1 1 0],[0 0 1 1],c1);patch([0 1 1 1-e 1-e 0+e],[0 0 1 1-e 0+e 0+e],c2);patch([0 0 1 1-e 0+e 0+e],[0 1 1 1-e 1-e 0+e],c3);plot([0 1 1 0 0],[0 0 1 1 0]);disp('W');
  "b{1}" : Constant  Value=[-1.602083138791444039128464282839559018611907958984375;0.7645476388269971668165680966922082006931304931640625;0.2199408905882851705815284049094771035015583038330078125;0.327328444308449262312166183619410730898380279541015625;0.3659761543007533646232332102954387664794921875;1.4137309227524166299616581454756669700145721435546875]
      mask Display: e = 0.06;c1 = [120 150 230]/255;c2 = ([120 150 230]+0)/383;c3 = ([120 150 230]+128)/383;patch([0 1 1 0],[0 0 1 1],c1);patch([0 1 1 1-e 1-e 0+e],[0 0 1 1-e 0+e 0+e],c2);patch([0 0 1 1-e 0+e 0+e],[0 1 1 1-e 1-e 0+e],c3);plot([0 1 1 0 0],[0 0 1 1 0]);disp('b');
  netsum : Sum  Inputs=2  InputSameDT=on  SaturateOnIntegerOverflow=on  OutDataTypeStr=Inherit: Same as first input
      mask Display: e = 0.06;c1 = [120 150 230]/255;c2 = ([120 150 230]+0)/383;c3 = ([120 150 230]+128)/383;patch([0 1 1 0],[0 0 1 1],c1);patch([0 1 1 1-e 1-e 0+e],[0 0 1 1-e 0+e 0+e],c2);patch([0 0 1 1-e 0+e 0+e],[0 1 1 1-e 1-e 0+e],c3);plot([0 1 1 0 0],[0 0 1 1 0]);disp('+');
  tansig : neural/Transfer Functions/tansig
  "a{1}" : Outport  InitialOutput=[0;0;0;0;0;0]
      mask Display: e = 0.06;c1 = [120 230 180]/255;c2 = ([120 230 180]+0)/(256+128);c3 = ([120 230 180]+128)/(256+128);patch([0 1 1 0],[0 0 1 1],c1);patch([0 1 1 1-e 1-e 0+e],[0 0 1 1-e 0+e 0+e],c2);patch([0 0 1 1-e 0+e 0+e],[0 1 1 1-e 1-e 0+e],c3);plot([0 1 1 0 0],[0 0 1 1 0]);
  wires:
  tansig/1 -> "a{1}"/1
  netsum/1 -> tansig/1
  "b{1}"/1 -> netsum/2
  "IW{1,1}"/1("iz{1,1}") -> netsum/1
  Delays 1/1("pd{1,1}") -> "IW{1,1}"/1("pd{1,1}")
  "p{1}"/1 -> Delays 1/1("p{1}")

== system chris_3R_hsv_all_primitives/pacific_blue_hsv_tuning1/RGB to HSV to vel - pacific-blue1/Pacific_blue_sat_net/Layer 2 ==
  "a{1} " : Inport  PortDimensions=6
      mask Display: e = 0.06;c1 = [120 230 180]/255;c2 = ([120 230 180]+0)/(256+128);c3 = ([120 230 180]+128)/(256+128);patch([0 1 1 0],[0 0 1 1],c1);patch([0 1 1 1-e 1-e 0+e],[0 0 1 1-e 0+e 0+e],c2);patch([0 0 1 1-e 0+e 0+e],[0 1 1 1-e 1-e 0+e],c3);plot([0 1 1 0 0],[0 0 1 1 0]);
  Delays 1 : Subsystem
      mask Display: e = 0.06;c1 = [120 150 230]/255;c2 = ([120 150 230]+0)/383;c3 = ([120 150 230]+128)/383;patch([0 1 1 0],[0 0 1 1],c1);patch([0 1 1 1-e 1-e 0+e],[0 0 1 1-e 0+e 0+e],c2);patch([0 0 1 1-e 0+e 0+e],[0 1 1 1-e 1-e 0+e],c3);plot([0 1 1 0 0],[0 0 1 1 0]);disp('0');
  "LW{2,1}" : Subsystem
      mask Display: e = 0.06;c1 = [120 150 230]/255;c2 = ([120 150 230]+0)/383;c3 = ([120 150 230]+128)/383;patch([0 1 1 0],[0 0 1 1],c1);patch([0 1 1 1-e 1-e 0+e],[0 0 1 1-e 0+e 0+e],c2);patch([0 0 1 1-e 0+e 0+e],[0 1 1 1-e 1-e 0+e],c3);plot([0 1 1 0 0],[0 0 1 1 0]);disp('W');
  "b{2}" : Constant  Value=[2.166919279225384631359929699101485311985015869140625;-0.5959275825915544277933122430113144218921661376953125;-1.0312953188054090336578383357846178114414215087890625;-1.064633194018286044268961632042191922664642333984375]
      mask Display: e = 0.06;c1 = [120 150 230]/255;c2 = ([120 150 230]+0)/383;c3 = ([120 150 230]+128)/383;patch([0 1 1 0],[0 0 1 1],c1);patch([0 1 1 1-e 1-e 0+e],[0 0 1 1-e 0+e 0+e],c2);patch([0 0 1 1-e 0+e 0+e],[0 1 1 1-e 1-e 0+e],c3);plot([0 1 1 0 0],[0 0 1 1 0]);disp('b');
  netsum : Sum  Inputs=2  InputSameDT=on  SaturateOnIntegerOverflow=on  OutDataTypeStr=Inherit: Same as first input
      mask Display: e = 0.06;c1 = [120 150 230]/255;c2 = ([120 150 230]+0)/383;c3 = ([120 150 230]+128)/383;patch([0 1 1 0],[0 0 1 1],c1);patch([0 1 1 1-e 1-e 0+e],[0 0 1 1-e 0+e 0+e],c2);patch([0 0 1 1-e 0+e 0+e],[0 1 1 1-e 1-e 0+e],c3);plot([0 1 1 0 0],[0 0 1 1 0]);disp('+');
  tansig : neural/Transfer Functions/tansig
  "a{2}" : Outport  InitialOutput=[0;0;0;0]
      mask Display: e = 0.06;c1 = [120 230 180]/255;c2 = ([120 230 180]+0)/(256+128);c3 = ([120 230 180]+128)/(256+128);patch([0 1 1 0],[0 0 1 1],c1);patch([0 1 1 1-e 1-e 0+e],[0 0 1 1-e 0+e 0+e],c2);patch([0 0 1 1-e 0+e 0+e],[0 1 1 1-e 1-e 0+e],c3);plot([0 1 1 0 0],[0 0 1 1 0]);
  wires:
  tansig/1 -> "a{2}"/1
  netsum/1 -> tansig/1
  "b{2}"/1 -> netsum/2
  "LW{2,1}"/1("lz{2,1}") -> netsum/1
  Delays 1/1("pd{2,1}") -> "LW{2,1}"/1("ad{2,1}")
  "a{1} "/1 -> Delays 1/1("p{2}")

== system chris_3R_hsv_all_primitives/pacific_blue_hsv_tuning1/RGB to HSV to vel - pacific-blue1/Pacific_blue_sat_net/Layer 3 ==
  "a{2} " : Inport  PortDimensions=4
      mask Display: e = 0.06;c1 = [120 230 180]/255;c2 = ([120 230 180]+0)/(256+128);c3 = ([120 230 180]+128)/(256+128);patch([0 1 1 0],[0 0 1 1],c1);patch([0 1 1 1-e 1-e 0+e],[0 0 1 1-e 0+e 0+e],c2);patch([0 0 1 1-e 0+e 0+e],[0 1 1 1-e 1-e 0+e],c3);plot([0 1 1 0 0],[0 0 1 1 0]);
  Delays 1 : Subsystem
      mask Display: e = 0.06;c1 = [120 150 230]/255;c2 = ([120 150 230]+0)/383;c3 = ([120 150 230]+128)/383;patch([0 1 1 0],[0 0 1 1],c1);patch([0 1 1 1-e 1-e 0+e],[0 0 1 1-e 0+e 0+e],c2);patch([0 0 1 1-e 0+e 0+e],[0 1 1 1-e 1-e 0+e],c3);plot([0 1 1 0 0],[0 0 1 1 0]);disp('0');
  "LW{3,2}" : Subsystem
      mask Display: e = 0.06;c1 = [120 150 230]/255;c2 = ([120 150 230]+0)/383;c3 = ([120 150 230]+128)/383;patch([0 1 1 0],[0 0 1 1],c1);patch([0 1 1 1-e 1-e 0+e],[0 0 1 1-e 0+e 0+e],c2);patch([0 0 1 1-e 0+e 0+e],[0 1 1 1-e 1-e 0+e],c3);plot([0 1 1 0 0],[0 0 1 1 0]);disp('W');
  "b{3}" : Constant  Value=[-0.7762294419301627446117208819487132132053375244140625;-1.9889324458139985285498596567776985466480255126953125]
      mask Display: e = 0.06;c1 = [120 150 230]/255;c2 = ([120 150 230]+0)/383;c3 = ([120 150 230]+128)/383;patch([0 1 1 0],[0 0 1 1],c1);patch([0 1 1 1-e 1-e 0+e],[0 0 1 1-e 0+e 0+e],c2);patch([0 0 1 1-e 0+e 0+e],[0 1 1 1-e 1-e 0+e],c3);plot([0 1 1 0 0],[0 0 1 1 0]);disp('b');
  netsum : Sum  Inputs=2  InputSameDT=on  SaturateOnIntegerOverflow=on  OutDataTypeStr=Inherit: Same as first input
      mask Display: e = 0.06;c1 = [120 150 230]/255;c2 = ([120 150 230]+0)/383;c3 = ([120 150 230]+128)/383;patch([0 1 1 0],[0 0 1 1],c1);patch([0 1 1 1-e 1-e 0+e],[0 0 1 1-e 0+e 0+e],c2);patch([0 0 1 1-e 0+e 0+e],[0 1 1 1-e 1-e 0+e],c3);plot([0 1 1 0 0],[0 0 1 1 0]);disp('+');
  tansig : neural/Transfer Functions/tansig
  "a{3}" : Outport  InitialOutput=[0;0]
      mask Display: e = 0.06;c1 = [120 230 180]/255;c2 = ([120 230 180]+0)/(256+128);c3 = ([120 230 180]+128)/(256+128);patch([0 1 1 0],[0 0 1 1],c1);patch([0 1 1 1-e 1-e 0+e],[0 0 1 1-e 0+e 0+e],c2);patch([0 0 1 1-e 0+e 0+e],[0 1 1 1-e 1-e 0+e],c3);plot([0 1 1 0 0],[0 0 1 1 0]);
  wires:
  tansig/1 -> "a{3}"/1
  netsum/1 -> tansig/1
  "b{3}"/1 -> netsum/2
  "LW{3,2}"/1("lz{3,2}") -> netsum/1
  Delays 1/1("pd{3,2}") -> "LW{3,2}"/1("ad{3,2}")
  "a{2} "/1 -> Delays 1/1("p{3}")

== system chris_3R_hsv_all_primitives/pacific_blue_hsv_tuning1/RGB to HSV to vel - pacific-blue1/Pacific_blue_sat_net/Layer 4 ==
  "a{3} " : Inport  PortDimensions=2
      mask Display: e = 0.06;c1 = [120 230 180]/255;c2 = ([120 230 180]+0)/(256+128);c3 = ([120 230 180]+128)/(256+128);patch([0 1 1 0],[0 0 1 1],c1);patch([0 1 1 1-e 1-e 0+e],[0 0 1 1-e 0+e 0+e],c2);patch([0 0 1 1-e 0+e 0+e],[0 1 1 1-e 1-e 0+e],c3);plot([0 1 1 0 0],[0 0 1 1 0]);
  Delays 1 : Subsystem
      mask Display: e = 0.06;c1 = [120 150 230]/255;c2 = ([120 150 230]+0)/383;c3 = ([120 150 230]+128)/383;patch([0 1 1 0],[0 0 1 1],c1);patch([0 1 1 1-e 1-e 0+e],[0 0 1 1-e 0+e 0+e],c2);patch([0 0 1 1-e 0+e 0+e],[0 1 1 1-e 1-e 0+e],c3);plot([0 1 1 0 0],[0 0 1 1 0]);disp('0');
  "LW{4,3}" : Subsystem
      mask Display: e = 0.06;c1 = [120 150 230]/255;c2 = ([120 150 230]+0)/383;c3 = ([120 150 230]+128)/383;patch([0 1 1 0],[0 0 1 1],c1);patch([0 1 1 1-e 1-e 0+e],[0 0 1 1-e 0+e 0+e],c2);patch([0 0 1 1-e 0+e 0+e],[0 1 1 1-e 1-e 0+e],c3);plot([0 1 1 0 0],[0 0 1 1 0]);disp('W');
  "b{4}" : Constant  Value=0.1279206937254931675251867773113190196454524993896484375
      mask Display: e = 0.06;c1 = [120 150 230]/255;c2 = ([120 150 230]+0)/383;c3 = ([120 150 230]+128)/383;patch([0 1 1 0],[0 0 1 1],c1);patch([0 1 1 1-e 1-e 0+e],[0 0 1 1-e 0+e 0+e],c2);patch([0 0 1 1-e 0+e 0+e],[0 1 1 1-e 1-e 0+e],c3);plot([0 1 1 0 0],[0 0 1 1 0]);disp('b');
  netsum : Sum  Inputs=2  InputSameDT=on  SaturateOnIntegerOverflow=on  OutDataTypeStr=Inherit: Same as first input
      mask Display: e = 0.06;c1 = [120 150 230]/255;c2 = ([120 150 230]+0)/383;c3 = ([120 150 230]+128)/383;patch([0 1 1 0],[0 0 1 1],c1);patch([0 1 1 1-e 1-e 0+e],[0 0 1 1-e 0+e 0+e],c2);patch([0 0 1 1-e 0+e 0+e],[0 1 1 1-e 1-e 0+e],c3);plot([0 1 1 0 0],[0 0 1 1 0]);disp('+');
  purelin : neural/Transfer Functions/purelin
  "a{4}" : Outport  InitialOutput=0
      mask Display: e = 0.06;c1 = [120 230 180]/255;c2 = ([120 230 180]+0)/(256+128);c3 = ([120 230 180]+128)/(256+128);patch([0 1 1 0],[0 0 1 1],c1);patch([0 1 1 1-e 1-e 0+e],[0 0 1 1-e 0+e 0+e],c2);patch([0 0 1 1-e 0+e 0+e],[0 1 1 1-e 1-e 0+e],c3);plot([0 1 1 0 0],[0 0 1 1 0]);
  wires:
  purelin/1 -> "a{4}"/1
  netsum/1 -> purelin/1
  "b{4}"/1 -> netsum/2
  "LW{4,3}"/1("lz{4,3}") -> netsum/1
  Delays 1/1("pd{4,3}") -> "LW{4,3}"/1("ad{4,3}")
  "a{3} "/1 -> Delays 1/1("p{4}")

== system chris_3R_hsv_all_primitives/pacific_blue_hsv_tuning1/RGB to HSV to vel - pacific-blue1/Pacific_blue_sat_net/Process Input 1 ==
  x : Inport  PortDimensions=7
      mask Display: e = 0.06;c1 = [120 230 180]/255;c2 = ([120 230 180]+0)/(256+128);c3 = ([120 230 180]+128)/(256+128);patch([0 1 1 0],[0 0 1 1],c1);patch([0 1 1 1-e 1-e 0+e],[0 0 1 1-e 0+e 0+e],c2);patch([0 0 1 1-e 0+e 0+e],[0 1 1 1-e 1-e 0+e],c3);plot([0 1 1 0 0],[0 0 1 1 0]);
  mapminmax : neural/Processing Functions/mapminmax  xmin=[-1;-1;-1;-1;-1;-0.839547345332068650769485884666;-0.607398217245419425047714412358]  xmax=[1;1;0.930903564414069739640922307444;0.924282590650705282442345378513;0.999480983360986119379276715335;1;1]  ymin=-1  ymax=1
  p : Outport  PortDimensions=7
      mask Display: e = 0.06;c1 = [120 230 180]/255;c2 = ([120 230 180]+0)/(256+128);c3 = ([120 230 180]+128)/(256+128);patch([0 1 1 0],[0 0 1 1],c1);patch([0 1 1 1-e 1-e 0+e],[0 0 1 1-e 0+e 0+e],c2);patch([0 0 1 1-e 0+e 0+e],[0 1 1 1-e 1-e 0+e],c3);plot([0 1 1 0 0],[0 0 1 1 0]);
  wires:
  mapminmax/1 -> p/1
  x/1 -> mapminmax/1

== system chris_3R_hsv_all_primitives/pacific_blue_hsv_tuning1/RGB to HSV to vel - pacific-blue1/Pacific_blue_sat_net/Process Output 1 ==
  a : Inport  PortDimensions=1
      mask Display: e = 0.06;c1 = [120 230 180]/255;c2 = ([120 230 180]+0)/(256+128);c3 = ([120 230 180]+128)/(256+128);patch([0 1 1 0],[0 0 1 1],c1);patch([0 1 1 1-e 1-e 0+e],[0 0 1 1-e 0+e 0+e],c2);patch([0 0 1 1-e 0+e 0+e],[0 1 1 1-e 1-e 0+e],c3);plot([0 1 1 0 0],[0 0 1 1 0]);
  mapminmax_reverse : neural/Processing Functions/mapminmax_reverse  xmin=-0.625  xmax=0.958399999999999918642856755469  ymin=-1  ymax=1
  y : Outport  PortDimensions=1
      mask Display: e = 0.06;c1 = [120 230 180]/255;c2 = ([120 230 180]+0)/(256+128);c3 = ([120 230 180]+128)/(256+128);patch([0 1 1 0],[0 0 1 1],c1);patch([0 1 1 1-e 1-e 0+e],[0 0 1 1-e 0+e 0+e],c2);patch([0 0 1 1-e 0+e 0+e],[0 1 1 1-e 1-e 0+e],c3);plot([0 1 1 0 0],[0 0 1 1 0]);
  wires:
  mapminmax_reverse/1 -> y/1
  a/1 -> mapminmax_reverse/1

== system chris_3R_hsv_all_primitives/pacific_blue_hsv_tuning1/RGB to HSV to vel - pacific-blue1/pacific_blue_hue_net/Layer 1 ==
  "p{1}" : Inport  PortDimensions=7
      mask Display: e = 0.06;c1 = [120 230 180]/255;c2 = ([120 230 180]+0)/(256+128);c3 = ([120 230 180]+128)/(256+128);patch([0 1 1 0],[0 0 1 1],c1);patch([0 1 1 1-e 1-e 0+e],[0 0 1 1-e 0+e 0+e],c2);patch([0 0 1 1-e 0+e 0+e],[0 1 1 1-e 1-e 0+e],c3);plot([0 1 1 0 0],[0 0 1 1 0]);
  Delays 1 : Subsystem
      mask Display: e = 0.06;c1 = [120 150 230]/255;c2 = ([120 150 230]+0)/383;c3 = ([120 150 230]+128)/383;patch([0 1 1 0],[0 0 1 1],c1);patch([0 1 1 1-e 1-e 0+e],[0 0 1 1-e 0+e 0+e],c2);patch([0 0 1 1-e 0+e 0+e],[0 1 1 1-e 1-e 0+e],c3);plot([0 1 1 0 0],[0 0 1 1 0]);disp('0');
  "IW{1,1}" : Subsystem
      mask Display: e = 0.06;c1 = [120 150 230]/255;c2 = ([120 150 230]+0)/383;c3 = ([120 150 230]+128)/383;patch([0 1 1 0],[0 0 1 1],c1);patch([0 1 1 1-e 1-e 0+e],[0 0 1 1-e 0+e 0+e],c2);patch([0 0 1 1-e 0+e 0+e],[0 1 1 1-e 1-e 0+e],c3);plot([0 1 1 0 0],[0 0 1 1 0]);disp('W');
  "b{1}" : Constant  Value=[0.369455181931211129597869557983358390629291534423828125;1.0513287794666699159762401905027218163013458251953125;-3.94777081983249455987561304937116801738739013671875;0.341630987749958148214091124827973544597625732421875;1.1998921930017889536657094140537083148956298828125]
      mask Display: e = 0.06;c1 = [120 150 230]/255;c2 = ([120 150 230]+0)/383;c3 = ([120 150 230]+128)/383;patch([0 1 1 0],[0 0 1 1],c1);patch([0 1 1 1-e 1-e 0+e],[0 0 1 1-e 0+e 0+e],c2);patch([0 0 1 1-e 0+e 0+e],[0 1 1 1-e 1-e 0+e],c3);plot([0 1 1 0 0],[0 0 1 1 0]);disp('b');
  netsum : Sum  Inputs=2  InputSameDT=on  SaturateOnIntegerOverflow=on  OutDataTypeStr=Inherit: Same as first input
      mask Display: e = 0.06;c1 = [120 150 230]/255;c2 = ([120 150 230]+0)/383;c3 = ([120 150 230]+128)/383;patch([0 1 1 0],[0 0 1 1],c1);patch([0 1 1 1-e 1-e 0+e],[0 0 1 1-e 0+e 0+e],c2);patch([0 0 1 1-e 0+e 0+e],[0 1 1 1-e 1-e 0+e],c3);plot([0 1 1 0 0],[0 0 1 1 0]);disp('+');
  tansig : neural/Transfer Functions/tansig
  "a{1}" : Outport  InitialOutput=[0;0;0;0;0]
      mask Display: e = 0.06;c1 = [120 230 180]/255;c2 = ([120 230 180]+0)/(256+128);c3 = ([120 230 180]+128)/(256+128);patch([0 1 1 0],[0 0 1 1],c1);patch([0 1 1 1-e 1-e 0+e],[0 0 1 1-e 0+e 0+e],c2);patch([0 0 1 1-e 0+e 0+e],[0 1 1 1-e 1-e 0+e],c3);plot([0 1 1 0 0],[0 0 1 1 0]);
  wires:
  "p{1}"/1 -> Delays 1/1("p{1}")
  Delays 1/1("pd{1,1}") -> "IW{1,1}"/1("pd{1,1}")
  "IW{1,1}"/1("iz{1,1}") -> netsum/1
  "b{1}"/1 -> netsum/2
  netsum/1 -> tansig/1
  tansig/1 -> "a{1}"/1
